simulink model "car_model_with_controller"  (R2020b)
settings: Solver=ode45  StartTime=0.0  StopTime=50  RelTol=1e-3
values from neighbouring files (symbols this model uses):
  N = length(traj.tSamples)    [tracking_accel.m]
  R = @(theta) [cos(theta),sin(theta),0;-sin(theta),cos(theta),0;0,0,1]    [local_error.m]
  T = traj.tSamples(2)    [tracking_accel.m]
undefined symbols (not defined in the file or in its folder): d, J, Kb, kd, ki, kp, Kt, l, L, m, r, theta_init, x_init, y_init
libraries: pid_lib x2
settings Model: Creator=Tiago  LastModifiedBy=francisco
settings DebuggingCC: SFMachineParentedDataDiag=error  UnderSpecifiedDimensionMsg=warning

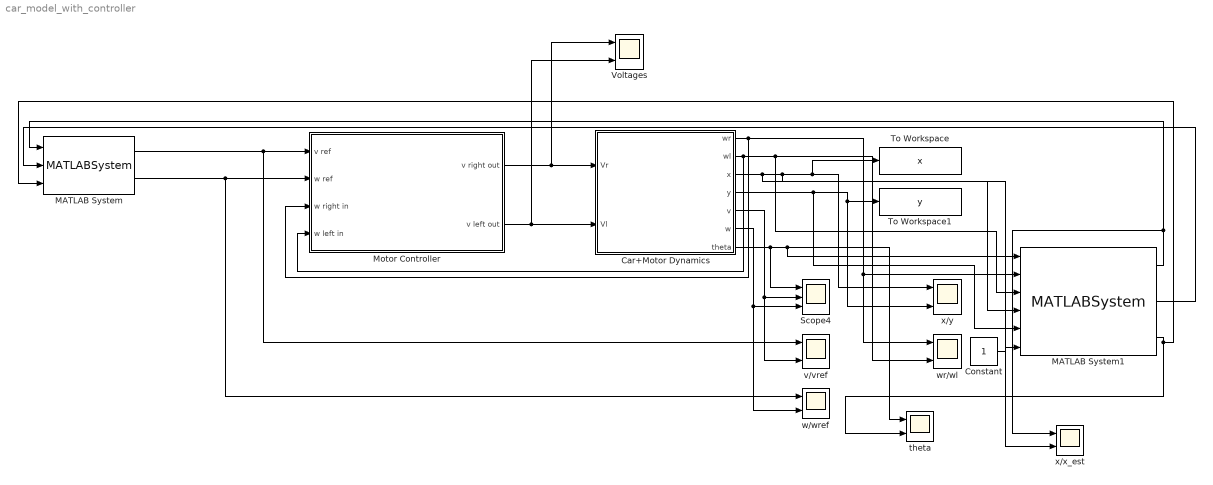
== system car_model_with_controller ==
  Car+Motor Dynamics : Subsystem
  Constant : Constant
  MATLAB System : MATLABSystem  System=kin_controller  traj=trajectory  OffsetTime=0.0  SampleTime=T  useKinematicModel=false  SimulateUsing=Code generation
      mask Type: kin_controller
      mask Display:
      | disp('kin_controller');
      | port_label('input',1,'x');
      | port_label('input',2,'y');
      | port_label('input',3,'theta');
      | port_label('output',1,'v');
      | port_label('output',2,'omega');
  MATLAB System1 : MATLABSystem  System=navigation  initial_x=x_init  initial_y=y_init  initial_theta=theta_init  q_gain=0.01  r_gain=0.001  OffsetTime=0.0  SampleTime=0.001  position_noise=2  orientation_noise=0.01  angular_speed_noise=0.01  SimulateUsing=Code generation
      mask Type: navigation
      mask Display:
      | disp('navigation');
      | port_label('input',1,'theta_measured');
      | port_label('input',2,'omega_r');
      | port_label('input',3,'omega_l');
      | port_label('input',4,'x_real');
      | port_label('input',5,'y_real');
      | port_label('input',6,'GPS');
      | port_label('output',1,'x');
      | port_label('output',2,'y');
      | port_label('output',3,'theta');
  Motor Controller : Subsystem
  Scope4 : Scope  NumInputPorts=3
  To Workspace : ToWorkspace  VariableName=x  SaveFormat=Timeseries  SampleTime=-1
  To Workspace1 : ToWorkspace  VariableName=y  SaveFormat=Timeseries  SampleTime=-1
  Voltages : Scope  NumInputPorts=2
  theta : Scope  NumInputPorts=2
  v/vref : Scope  NumInputPorts=2
  w/wref : Scope  NumInputPorts=2
  wr/wl : Scope  NumInputPorts=2
  x/x_est : Scope  NumInputPorts=2
  x/y : Scope  NumInputPorts=2
  wires:
  Motor Controller/2(v left out) -> Voltages/2, Car+Motor Dynamics/2(Vl)
  Motor Controller/1(v right out) -> Voltages/1, Car+Motor Dynamics/1(Vr)
  Car+Motor Dynamics/2(wl) -> Motor Controller/4(w left in), MATLAB System1/3, wr/wl/2
  Car+Motor Dynamics/1(wr) -> Motor Controller/3(w right in), MATLAB System1/2, wr/wl/1
  Car+Motor Dynamics/5(v) -> v/vref/2, Scope4/2
  Car+Motor Dynamics/6(w) -> w/wref/2, Scope4/3
  MATLAB System/1 -> Motor Controller/1(v ref), v/vref/1
  MATLAB System/2 -> w/wref/1, Motor Controller/2(w ref)
  Car+Motor Dynamics/7(theta) -> MATLAB System1/1, theta/1, Scope4/1
  Car+Motor Dynamics/3(x) -> x/x_est/2, MATLAB System1/4, x/y/1, To Workspace/1
  Car+Motor Dynamics/4(y) -> MATLAB System1/5, x/y/2, To Workspace1/1
  MATLAB System1/1 -> x/x_est/1, MATLAB System/1
  MATLAB System1/2 -> MATLAB System/2
  MATLAB System1/3 -> theta/2, MATLAB System/3
  Constant/1 -> MATLAB System1/6

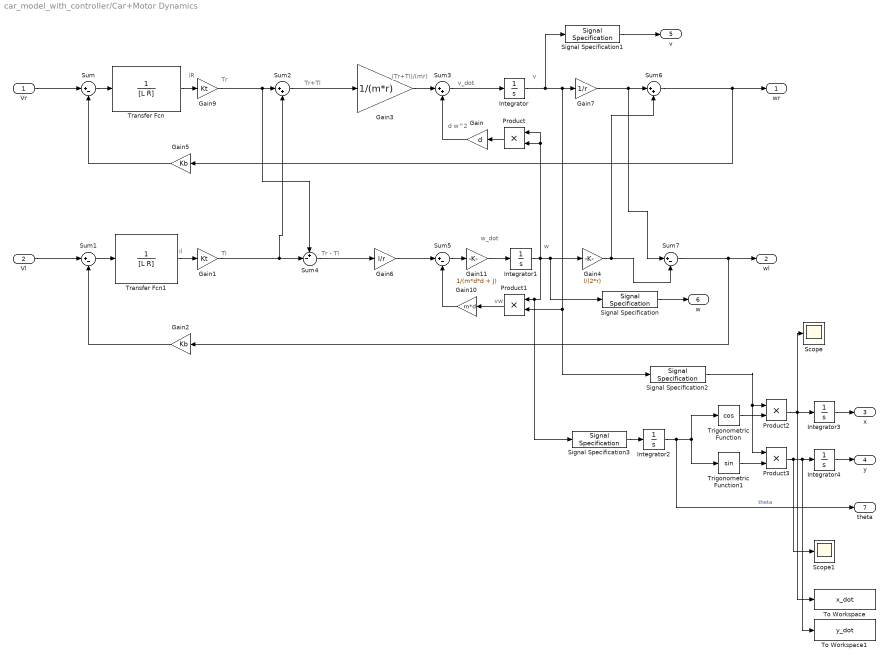
== system car_model_with_controller/Car+Motor Dynamics ==
  note: Tr - Tl
  note: vw
  note: d w^2
  note: v
  note: il
  note: Tr+Tl
  note: w_dot
  note: Tr
  note: (Tr+Tl)/(mr)
  note: v_dot
  note: w
  note: iR
  note: Tl
  Vr : Inport
  Vl : Inport  Port=2
  Gain : Gain  Gain=d
  Gain1 : Gain  Gain=Kt
  Gain10 : Gain  Gain=m*d
  Gain11 : Gain  Gain=1/(m*d*d + J)
  Gain2 : Gain  Gain=Kb
  Gain3 : Gain  Gain=1/(m*r)
  Gain4 : Gain  Gain=l/(2*r)
  Gain5 : Gain  Gain=Kb
  Gain6 : Gain  Gain=l/r
  Gain7 : Gain  Gain=1/r
  Gain9 : Gain  Gain=Kt
  Integrator : Integrator
  Integrator1 : Integrator
  Integrator2 : Integrator  InitialCondition=theta_init
  Integrator3 : Integrator  InitialCondition=x_init
  Integrator4 : Integrator  InitialCondition=y_init
  Product{,1..3} (4 alike) : Product
  Scope : Scope
  Scope1 : Scope
  Signal Specification{,1..3} (4 alike) : SignalSpecification  Dimensions=1
  Sum{,1,5,7} (4 alike) : Sum  Inputs=|+-
  Sum2 : Sum  Inputs=|++
  Sum3 : Sum  Inputs=|++
  Sum4 : Sum  Inputs=+-|
  Sum6 : Sum  Inputs=|++
  To Workspace : ToWorkspace  VariableName=x_dot  SaveFormat=Timeseries  SampleTime=-1
  To Workspace1 : ToWorkspace  VariableName=y_dot  SaveFormat=Timeseries  SampleTime=-1
  Transfer Fcn : TransferFcn  Denominator=[L R]
  Transfer Fcn1 : TransferFcn  Denominator=[L R]
  Trigonometric Function : Trigonometry  Operator=cos
  Trigonometric Function1 : Trigonometry
  wr : Outport
  wl : Outport  Port=2
  x : Outport  Port=3
  y : Outport  Port=4
  v : Outport  Port=5
  w : Outport  Port=6
  theta : Outport  Port=7
  wires:
  Gain/1 -> Sum3/2
  Sum7/1 -> Gain2/1, wl/1
  Product1/1 -> Gain10/1
  Sum1/1 -> Transfer Fcn1/1
  Sum6/1 -> wr/1, Gain5/1
  Product/1 -> Gain/1
  Sum5/1 -> Gain11/1
  Gain10/1 -> Sum5/2
  Gain3/1 -> Sum3/1
  Gain11/1 -> Integrator1/1
  Sum2/1 -> Gain3/1
  Vl/1 -> Sum1/1
  Sum3/1 -> Integrator/1
  Gain6/1 -> Sum5/1
  Gain4/1 -> Sum7/2, Sum6/2
  Transfer Fcn1/1 -> Gain1/1
  Sum/1 -> Transfer Fcn/1
  Vr/1 -> Sum/1
  Integrator1/1 -> Signal Specification3/1, Product1/1, Signal Specification/1, Gain4/1, Product/1, Product/2
  Transfer Fcn/1 -> Gain9/1
  Integrator2/1 -> theta/1, Trigonometric Function1/1, Trigonometric Function/1  "theta"
  Trigonometric Function/1 -> Product2/2
  Trigonometric Function1/1 -> Product3/2
  Product3/1 -> Scope1/1, To Workspace1/1, Integrator4/1
  Product2/1 -> To Workspace/1, Integrator3/1, Scope/1
  Integrator3/1 -> x/1
  Integrator4/1 -> y/1
  Sum4/1 -> Gain6/1
  Gain1/1 -> Sum2/2, Sum4/2
  Gain9/1 -> Sum4/1, Sum2/1
  Gain5/1 -> Sum/2
  Gain2/1 -> Sum1/2
  Gain7/1 -> Sum6/1, Sum7/1
  Integrator/1 -> Signal Specification1/1, Gain7/1, Signal Specification2/1, Product1/2
  Signal Specification/1 -> w/1
  Signal Specification1/1 -> v/1
  Signal Specification2/1 -> Product3/1, Product2/1
  Signal Specification3/1 -> Integrator2/1

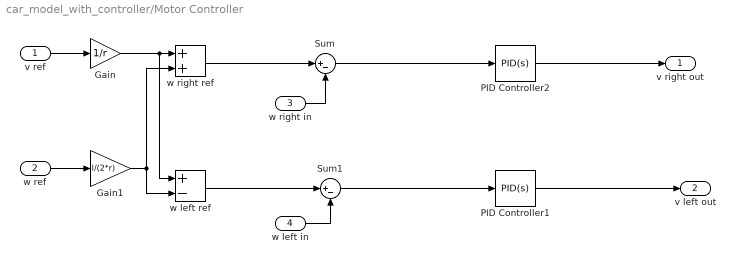
== system car_model_with_controller/Motor Controller ==
  v ref : Inport
  w ref : Inport  Port=2
  w right in : Inport  Port=3
  w left in : Inport  Port=4
  Gain : Gain  Gain=1/r
  Gain1 : Gain  Gain=l/(2*r)
  PID Controller1 : pid_lib/PID Controller  Controller=PID  Form=Parallel  TimeDomain=Continuous-time  UseExternalTs=off  SampleTime=-1  IntegratorMethod=Forward Euler  FilterMethod=Forward Euler  ControllerParametersSource=internal  P=kp  I=ki  D=kd  UseFilter=on  N=105296.504032148  TunerSelectOption=Transfer Function Based (PID Tuner App)  InitialConditionSource=internal  InitialConditionForIntegrator=0  InitialConditionForFilter=0  DifferentiatorICPrevScaledInput=0  ExternalReset=none  TrackingMode=off  Kt=1  LimitOutput=off  SatLimitsSource=internal  UpperSaturationLimit=inf  LowerSaturationLimit=-inf  LinearizeAsGain=on  AntiWindupMode=none  Kb=1  POutMin=[]  POutMax=[]  IOutMin=[]  IOutMax=[]  DOutMin=[]  DOutMax=[]  NOutMin=[]  NOutMax=[]  SumOutMin=[]  SumOutMax=[]  SaturationOutMin=[]  SaturationOutMax=[]  PParamMin=[]  PParamMax=[]  IParamMin=[]  IParamMax=[]  DParamMin=[]  DParamMax=[]  NParamMin=[]  NParamMax=[]  KbParamMin=[]  KbParamMax=[]  KtParamMin=[]  KtParamMax=[]  KbOutMin=[]  KbOutMax=[]  KtOutMin=[]  KtOutMax=[]  IntegratorOutMin=[]  IntegratorOutMax=[]  FilterOutMin=[]  FilterOutMax=[]  SumI1OutMin=[]  SumI1OutMax=[]  SumI2OutMin=[]  SumI2OutMax=[]  SumI3OutMin=[]  SumI3OutMax=[]  SumI4OutMin=[]  SumI4OutMax=[]  SumDOutMin=[]  SumDOutMax=[]  DifferentiatorOutMin=[]  DifferentiatorOutMax=[]  FilterDiffOutCoefMin=[]  FilterDiffOutCoefMax=[]  ReciprocalOutMin=[]  ReciprocalOutMax=[]  SumDenOutMin=[]  SumDenOutMax=[]  SumNumOutMin=[]  SumNumOutMax=[]  DivideOutMin=[]  DivideOutMax=[]  UdiffTsProdOutMin=[]  UdiffTsProdOutMax=[]  NTsProdOutMin=[]  NTsProdOutMax=[]  UintegralTsProdOutMin=[]  UintegralTsProdOutMax=[]  UngainTsProdOutMin=[]  UngainTsProdOutMax=[]  IntegratorContinuousStateAttributes=''  IntegratorStateMustResolveToSignalObject=off  IntegratorRTWStateStorageClass=Auto  FilterContinuousStateAttributes=''  FilterStateMustResolveToSignalObject=off  FilterRTWStateStorageClass=Auto  ParallelPVariant=InternalParameters  IdealPVariant=Disabled  IVariant=InternalParameters  DVariant=InternalParameters  IntegratorVariant=Continuous  SatVariant=Disabled  AWVariant=Passthrough  PCopyVariant=Disabled  TRVariant=Disabled  FdbkBlocksVariant=Forward  IdealPFdbkVariant=Disabled  SatFdbkVariant=Disabled  DerivativeFilterVariant=ContFilter  NVariant=InternalParameters  NCopyVariant=Disabled  FilterICVariant=InternalICsFilter  IntegratorICVariant=InternalICs  ExternalResetVariant=Disabled  TRSumVariant=Passthrough  SumFdbkVariant=Disabled  SumVariant=Sum_PID  TsampFilterVariant=InternalTs  TsampNgainVariant=Passthrough  TsampIntegralVariant=Passthrough  ExternalSaturationOutDataTypeStr=Inherit: Same as second input
  PID Controller2 : pid_lib/PID Controller  Controller=PID  Form=Parallel  TimeDomain=Continuous-time  UseExternalTs=off  SampleTime=-1  IntegratorMethod=Forward Euler  FilterMethod=Forward Euler  ControllerParametersSource=internal  P=ki  I=kp  D=kd  UseFilter=on  N=N  TunerSelectOption=Transfer Function Based (PID Tuner App)  InitialConditionSource=internal  InitialConditionForIntegrator=0  InitialConditionForFilter=0  DifferentiatorICPrevScaledInput=0  ExternalReset=none  TrackingMode=off  Kt=1  LimitOutput=off  SatLimitsSource=internal  UpperSaturationLimit=inf  LowerSaturationLimit=-inf  LinearizeAsGain=on  AntiWindupMode=none  Kb=1  POutMin=[]  POutMax=[]  IOutMin=[]  IOutMax=[]  DOutMin=[]  DOutMax=[]  NOutMin=[]  NOutMax=[]  SumOutMin=[]  SumOutMax=[]  SaturationOutMin=[]  SaturationOutMax=[]  PParamMin=[]  PParamMax=[]  IParamMin=[]  IParamMax=[]  DParamMin=[]  DParamMax=[]  NParamMin=[]  NParamMax=[]  KbParamMin=[]  KbParamMax=[]  KtParamMin=[]  KtParamMax=[]  KbOutMin=[]  KbOutMax=[]  KtOutMin=[]  KtOutMax=[]  IntegratorOutMin=[]  IntegratorOutMax=[]  FilterOutMin=[]  FilterOutMax=[]  SumI1OutMin=[]  SumI1OutMax=[]  SumI2OutMin=[]  SumI2OutMax=[]  SumI3OutMin=[]  SumI3OutMax=[]  SumI4OutMin=[]  SumI4OutMax=[]  SumDOutMin=[]  SumDOutMax=[]  DifferentiatorOutMin=[]  DifferentiatorOutMax=[]  FilterDiffOutCoefMin=[]  FilterDiffOutCoefMax=[]  ReciprocalOutMin=[]  ReciprocalOutMax=[]  SumDenOutMin=[]  SumDenOutMax=[]  SumNumOutMin=[]  SumNumOutMax=[]  DivideOutMin=[]  DivideOutMax=[]  UdiffTsProdOutMin=[]  UdiffTsProdOutMax=[]  NTsProdOutMin=[]  NTsProdOutMax=[]  UintegralTsProdOutMin=[]  UintegralTsProdOutMax=[]  UngainTsProdOutMin=[]  UngainTsProdOutMax=[]  IntegratorContinuousStateAttributes=''  IntegratorStateMustResolveToSignalObject=off  IntegratorRTWStateStorageClass=Auto  FilterContinuousStateAttributes=''  FilterStateMustResolveToSignalObject=off  FilterRTWStateStorageClass=Auto  ParallelPVariant=InternalParameters  IdealPVariant=Disabled  IVariant=InternalParameters  DVariant=InternalParameters  IntegratorVariant=Continuous  SatVariant=Disabled  AWVariant=Passthrough  PCopyVariant=Disabled  TRVariant=Disabled  FdbkBlocksVariant=Forward  IdealPFdbkVariant=Disabled  SatFdbkVariant=Disabled  DerivativeFilterVariant=ContFilter  NVariant=InternalParameters  NCopyVariant=Disabled  FilterICVariant=InternalICsFilter  IntegratorICVariant=InternalICs  ExternalResetVariant=Disabled  TRSumVariant=Passthrough  SumFdbkVariant=Disabled  SumVariant=Sum_PID  TsampFilterVariant=InternalTs  TsampNgainVariant=Passthrough  TsampIntegralVariant=Passthrough  ExternalSaturationOutDataTypeStr=Inherit: Same as second input
  Sum : Sum  Inputs=|+-
  Sum1 : Sum  Inputs=|+-
  w left ref : Sum  Inputs=+-
  w right ref : Sum
  v right out : Outport
  v left out : Outport  Port=2
  wires:
  v ref/1 -> Gain/1
  Gain/1 -> w right ref/1, w left ref/1
  Gain1/1 -> w right ref/2, w left ref/2
  w right ref/1 -> Sum/1
  w left ref/1 -> Sum1/1
  w right in/1 -> Sum/2
  w left in/1 -> Sum1/2
  Sum/1 -> PID Controller2/1
  Sum1/1 -> PID Controller1/1
  w ref/1 -> Gain1/1
  PID Controller2/1 -> v right out/1
  PID Controller1/1 -> v left out/1
